simulink model "FuelController"  (R2022a)
settings: Solver=ode1  StartTime=0.0  StopTime=40  FixedStep=0.01  RelTol=1e-3  EnableMultiTasking=on
InitFcn:
  | FuelSimFinalModParameters
undefined symbols (not defined in the file or in its folder): AFc, etac, KM, Nc, R, T, tauc, tauM, TL, Vd, Vi, Xc
settings Model: Creator=burl  LastModifiedBy=Chaitanya
settings SolverCC: AlgebraicLoopSolver=TrustRegion
settings DataIOCC: ReturnWorkspaceOutputs=off
settings OptimizationCC: LifeSpan=inf
settings DebuggingCC: UnconnectedInputMsg=warning  UnconnectedOutputMsg=warning  UnconnectedLineMsg=warning  SFUnexpectedBacktrackingDiag=warning  SFNoUnconditionalDefaultTransitionDiag=warning  SFExecutionAtInitializationDiag=none  SFMachineParentedDataDiag=warning  ArithmeticOperatorsInVariantConditions=warning
settings SFSimCC: SimUseLocalCustomCode=off  CustomCodeUndefinedFunction=UseInterfaceOnly
settings RTWCC: RTWUseLocalCustomCode=off
settings CodeAppCC: StateflowObjectComments=on
settings GRTTargetCC: TargetLangStandard=C89/C90 (ANSI)
settings ConfigComp: CovMetricSettings=dw  CovSaveCumulativeToWorkspaceVar=on  CovSaveSingleToWorkspaceVar=on  CovExternalEMLEnable=off

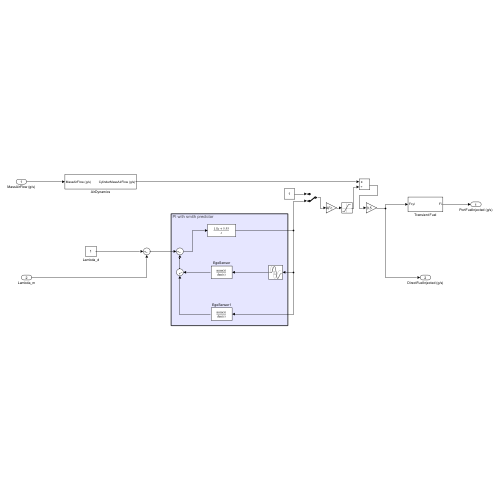
[thumbnail: Simulink's stored preview of the top-level diagram]
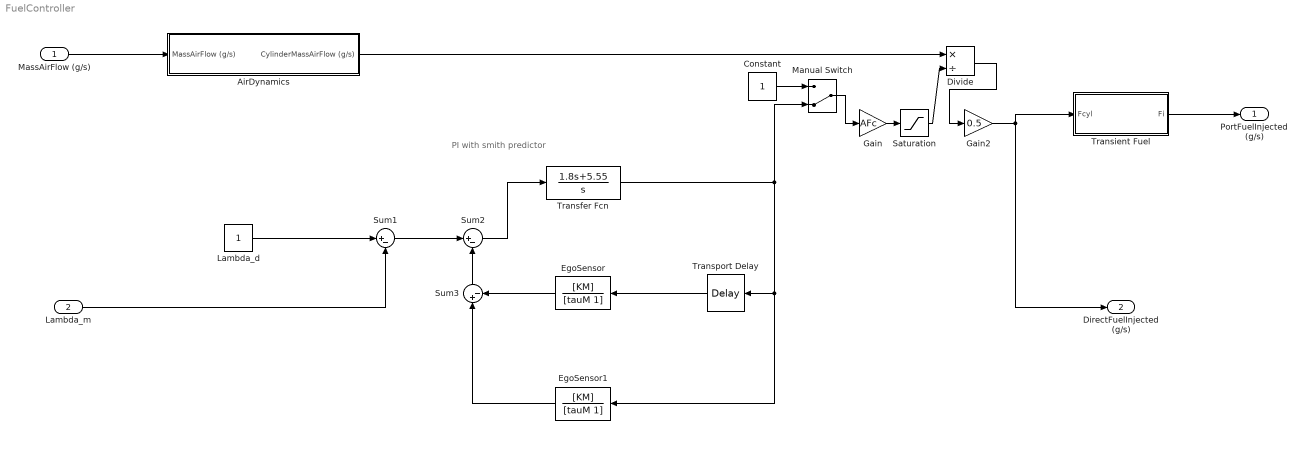
== system FuelController ==
  note: PI with smith predictor
  MassAirFlow (g/s) : Inport
  Lambda_m : Inport  Port=2
  AirDynamics : Subsystem
  Constant : Constant
  Divide : Product  Inputs=*/
  EgoSensor : TransferFcn  Numerator=[KM]  Denominator=[tauM 1]
  EgoSensor1 : TransferFcn  Numerator=[KM]  Denominator=[tauM 1]
  Gain : Gain  Gain=AFc
  Gain2 : Gain  Gain=0.5
  Lambda_d : Constant
  Manual Switch : ManualSwitch  CurrentSetting=0
  Saturation : Saturate  UpperLimit=1000000  LowerLimit=0.00005
  Sum1 : Sum  Inputs=|+-
  Sum2 : Sum  Inputs=|+-
  Sum3 : Sum  Inputs=|+-
  Transfer Fcn : TransferFcn  Numerator=[1.8 5.55]  Denominator=[1 0]
  Transient Fuel : Subsystem
  Transport Delay : TransportDelay  DelayTime=TL
  PortFuelInjected (g/s) : Outport  VectorParamsAs1DForOutWhenUnconnected=off
  DirectFuelInjected (g/s) : Outport  Port=2  VectorParamsAs1DForOutWhenUnconnected=off
  wires:
  MassAirFlow (g/s)/1 -> AirDynamics/1(MassAirFlow (g/s))
  Gain2/1 -> Transient Fuel/1(Fcyl), DirectFuelInjected (g/s)/1
  Sum1/1 -> Sum2/1
  Sum2/1 -> Transfer Fcn/1
  Transport Delay/1 -> EgoSensor/1
  EgoSensor/1 -> Sum3/2
  EgoSensor1/1 -> Sum3/1
  Sum3/1 -> Sum2/2
  Lambda_m/1 -> Sum1/2
  Lambda_d/1 -> Sum1/1
  AirDynamics/1(CylinderMassAirFlow (g/s)) -> Divide/1
  Gain/1 -> Saturation/1
  Saturation/1 -> Divide/2
  Divide/1 -> Gain2/1
  Transfer Fcn/1 -> Manual Switch/2, Transport Delay/1, EgoSensor1/1
  Constant/1 -> Manual Switch/1
  Manual Switch/1 -> Gain/1
  Transient Fuel/1(Fi) -> PortFuelInjected (g/s)/1

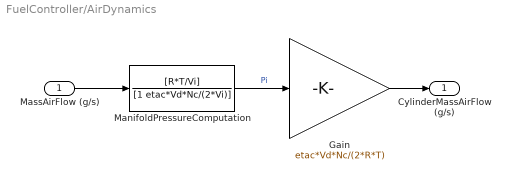
== system FuelController/AirDynamics ==
  MassAirFlow (g/s) : Inport
  Gain : Gain  Gain=etac*Vd*Nc/(2*R*T)
  ManifoldPressureComputation : TransferFcn  Numerator=[R*T/Vi]  Denominator=[1 etac*Vd*Nc/(2*Vi)]
  CylinderMassAirFlow (g/s) : Outport  VectorParamsAs1DForOutWhenUnconnected=off
  wires:
  MassAirFlow (g/s)/1 -> ManifoldPressureComputation/1
  ManifoldPressureComputation/1 -> Gain/1  "Pi"
  Gain/1 -> CylinderMassAirFlow (g/s)/1

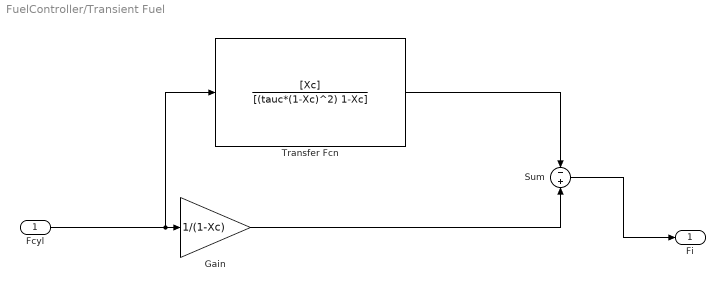
== system FuelController/Transient Fuel ==
  Fcyl : Inport
  Gain : Gain  Gain=1/(1-Xc)
  Sum : Sum  Inputs=-+
  Transfer Fcn : TransferFcn  Numerator=[Xc]  Denominator=[(tauc*(1-Xc)^2) 1-Xc]
  Fi : Outport
  wires:
  Fcyl/1 -> Transfer Fcn/1, Gain/1
  Transfer Fcn/1 -> Sum/1
  Gain/1 -> Sum/2
  Sum/1 -> Fi/1
